simulink model "PRACTICAIMULINK"  (R2020a)
settings: Solver=FixedStepAuto  StartTime=0.0  StopTime=2010.0  FixedStep=0.02  RelTol=1e-3
undefined symbols (not defined in the file or in its folder): A, B, C, D
settings Model: Creator=TJGO  LastModifiedBy=TJGO

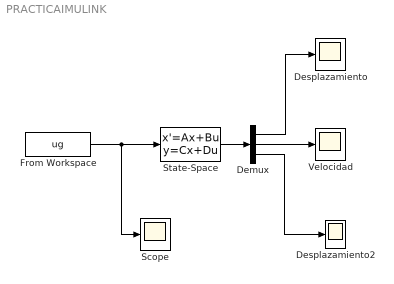
== system PRACTICAIMULINK ==
  Demux : Demux  Outputs=3
  Desplazamiento : Scope
  Desplazamiento2 : Scope
  From Workspace : FromWorkspace  VariableName=ug
  Scope : Scope
  State-Space : StateSpace  A=A  B=B  C=C  D=D  InitialCondition=0
  Velocidad : Scope
  wires:
  From Workspace/1 -> Scope/1, State-Space/1
  State-Space/1 -> Demux/1
  Demux/1 -> Desplazamiento/1
  Demux/2 -> Velocidad/1
  Demux/3 -> Desplazamiento2/1
